simulink model "bcdUpCounter"  (R2024a)
settings: Solver=VariableStepAuto  StartTime=0.0  StopTime=10.0  RelTol=1e-3
libraries: simulink_extras x5
settings Model: Creator=prath  LastModifiedBy=prath

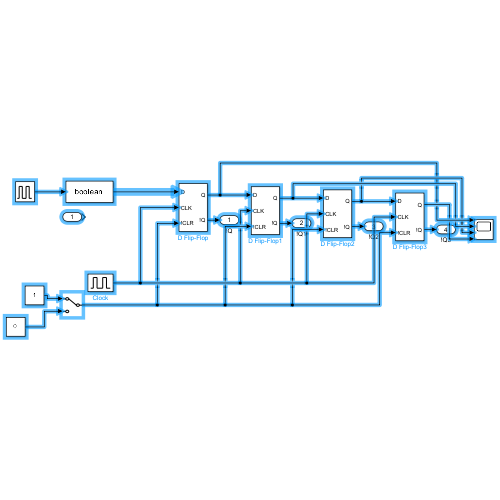
[thumbnail: Simulink's stored preview of the top-level diagram]
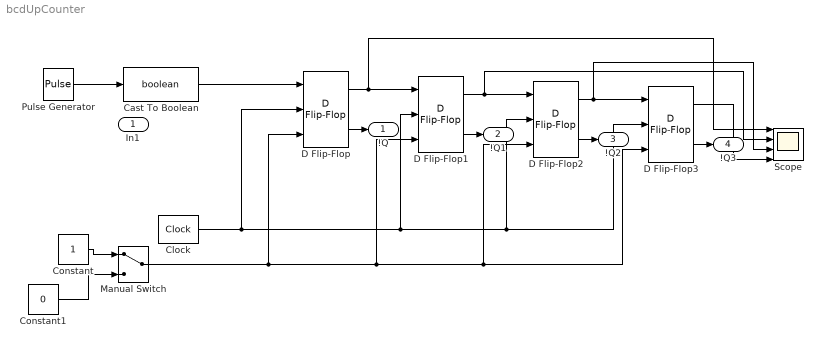
== system bcdUpCounter ==
  In1 : Inport
  Cast To Boolean : DataTypeConversion  OutDataTypeStr=boolean  SaturateOnIntegerOverflow=off  RndMeth=Floor
  Clock : simulink_extras/Flip Flops/Clock  period=1/2
  Constant : Constant  OutDataTypeStr=boolean
  Constant1 : Constant  Value=0  OutDataTypeStr=boolean
  D Flip-Flop{,1..3} (4 alike) : simulink_extras/Flip Flops/D Flip-Flop
  Manual Switch : ManualSwitch
  Pulse Generator : DiscretePulseGenerator  PulseType=Time based  Period=1  PulseWidth=50
  Scope : Scope  NumInputPorts=4
  !Q : Outport
  !Q1 : Outport  Port=2
  !Q2 : Outport  Port=3
  !Q3 : Outport  Port=4
  wires:
  D Flip-Flop2/2 -> !Q2/1
  Constant/1 -> Manual Switch/1
  D Flip-Flop3/1 -> Scope/4
  D Flip-Flop/2 -> !Q/1
  Clock/1 -> D Flip-Flop1/2, D Flip-Flop2/2, D Flip-Flop3/2, D Flip-Flop/2
  Pulse Generator/1 -> Cast To Boolean/1
  D Flip-Flop3/2 -> !Q3/1
  D Flip-Flop1/2 -> !Q1/1
  D Flip-Flop/1 -> Scope/1, D Flip-Flop1/1
  D Flip-Flop1/1 -> Scope/2, D Flip-Flop2/1
  Constant1/1 -> Manual Switch/2
  D Flip-Flop2/1 -> Scope/3, D Flip-Flop3/1
  Manual Switch/1 -> D Flip-Flop2/3, D Flip-Flop3/3, D Flip-Flop1/3, D Flip-Flop/3
  Cast To Boolean/1 -> D Flip-Flop/1
